simulink subsystem "AS_O2Input"  (R2022b)
settings: Solver=VariableStepAuto  StartTime=0.0  StopTime=10.0  RelTol=1e-3
undefined symbols (not defined in the file): O2_OutputDia
libraries: fl_lib x8, SimscapeFluids_lib x3, nesl_utility x3
settings Model: DefaultTestHarness=AS_O2Input_Test  Creator=CSN-Simulation  LastModifiedBy=MATLAB
settings DebuggingCC: UnconnectedInputMsg=warning  UnconnectedOutputMsg=warning  UnconnectedLineMsg=warning
settings ModelReferenceCC: EnableRefExpFcnMdlSchedulingChecks=on
settings RTWCC: DLArmComputeVersion=19.05

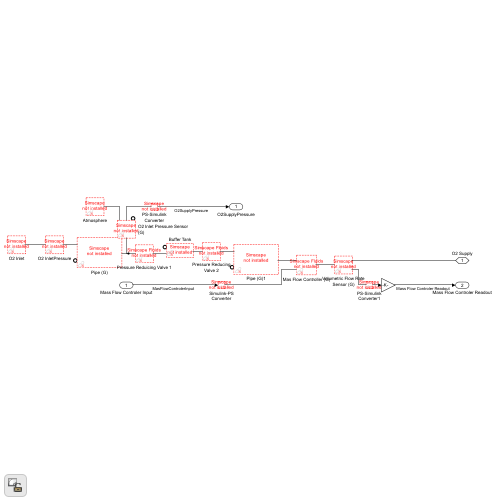
[thumbnail: Simulink's stored preview of the top-level diagram]
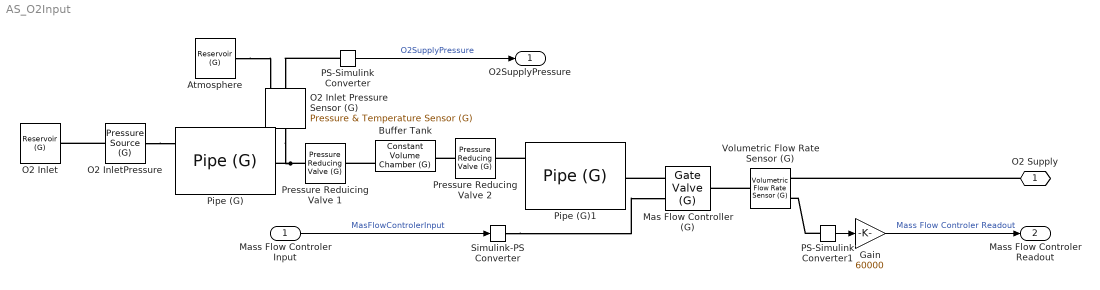
== system AS_O2Input ==
  Mass Flow Controler Input : Inport
  Atmosphere : fl_lib/Gas/Elements/Reservoir (G)  pressure_spec=foundation.enum.pressure_spec.atmospheric  reservoir_pressure=0.101325 MPa  reservoir_temperature=293.15 K  area_A=pi*(O2_OutputDia/2)^2 mm^2
  Buffer Tank : fl_lib/Gas/Elements/Constant Volume Chamber (G)  volume=O2_buffertank mm^3  num_ports=foundation.enum.num_ports.two  area_A=pi*(O2_OutputDia/2)^2 mm^2  area_B=pi*(O2_OutputDia/2)^2 mm^2  area_C=0.01 m^2  area_D=0.01 m^2  p_I_specify=off  p_I_priority=High  p_I=P_intermidiate Pa  p_I_nominal_specify=off  p_I_nominal_unit=MPa  p_I_nominal_value=1  T_I_specify=off  T_I_priority=High  T_I=T_room degC  T_I_nominal_specify=off  T_I_nominal_unit=K  T_I_nominal_value=1  rho_chamber_specify=off  rho_chamber_priority=None  rho_chamber=1.2 kg/m^3  rho_chamber_nominal_specify=off  rho_chamber_nominal_unit=kg/m^3  rho_chamber_nominal_value=1
      settings: InternalSimscapePortConfiguration="{\"Bottom\":[],\"Left\":[{\"id\":\"A\",\"label\":\"A\",\"type\":\"foundation.gas.gas\"},{\"id\":\"H\",\"label\":\"H\",\"type\":\"foundation.thermal.thermal\"}],\"Right\":[{\"id\":\"B\",\"label\":\"B\",\"type\":\"foundation.gas.gas\"}],\"Top\":[]}"
  Gain : Gain  Gain=60000
  Mas Flow Controller (G) : SimscapeFluids_lib/Gas/Valves & Orifices/Flow Control Valves/Gate Valve (G)  diam_orifice=O2_OutputDia-2 mm  x0=0  iso_cond_spec=fluids.gas.enum.flow_control_valve_spec.geometry  C_max=1.6 l/s/bar  B_crit=0.3  m=0.5  Cv_max=0.4  Kv_max=0.3  area_leak=1e-12 mm^2  area=pi*(O2_OutputDia/2)^2 mm^2  smoothing_factor=0  B_lam=0.999  T0=T_room degC  rho0=1.185 kg/m^3
      settings: InternalSimscapePortConfiguration="{\"Bottom\":[],\"Left\":[{\"id\":\"A\",\"label\":\"A\",\"type\":\"foundation.gas.gas\"},{\"id\":\"L\",\"label\":\"L\",\"type\":\"input\"}],\"Right\":[{\"id\":\"B\",\"label\":\"B\",\"type\":\"foundation.gas.gas\"}],\"Top\":[]}"
  O2 Inlet : fl_lib/Gas/Elements/Reservoir (G)  pressure_spec=foundation.enum.pressure_spec.atmospheric  reservoir_pressure=0.101325 MPa  reservoir_temperature=T_room degC  area_A=pi*(O2_OutputDia/2)^2 mm^2
  O2 Inlet Pressure Sensor (G) : fl_lib/Gas/Sensors/Pressure & Temperature Sensor (G)
      settings: InternalSimscapePortConfiguration="{\"Bottom\":[],\"Left\":[{\"id\":\"A\",\"label\":\"A\",\"type\":\"foundation.gas.gas\"}],\"Right\":[{\"id\":\"B\",\"label\":\"B\",\"type\":\"foundation.gas.gas\"},{\"id\":\"P\",\"label\":\"P\",\"type\":\"output\"},{\"id\":\"T\",\"label\":\"T\",\"type\":\"output\"}],\"Top\":[]}"
  O2 InletPressure : fl_lib/Gas/Sources/Pressure Source (G)  power_spec=foundation.enum.power_spec.isentropic  pressure_differential=P_inlet Pa  area_A=pi*(O2_OutputDia/2)^2 mm^2  area_B=pi*(O2_OutputDia/2)^2 mm^2
      settings: InternalSimscapePortConfiguration="{\"Bottom\":[],\"Left\":[{\"id\":\"A\",\"label\":\"A\",\"type\":\"foundation.gas.gas\"}],\"Right\":[{\"id\":\"B\",\"label\":\"B\",\"type\":\"foundation.gas.gas\"}],\"Top\":[]}"
  PS-Simulink Converter : nesl_utility/PS-Simulink Converter  PhysicalDomain=network_engine_domain  SubClassName=ps_output  LeftPortType=input  RightPortType=output  PseudoPeriodic=off  Frequencies=[]  Unit=Pa  AffineConversion=off
  PS-Simulink Converter1 : nesl_utility/PS-Simulink Converter  PhysicalDomain=network_engine_domain  SubClassName=ps_output  LeftPortType=input  RightPortType=output  PseudoPeriodic=off  Frequencies=[]  Unit=inherit  AffineConversion=off
  Pipe (G) : fl_lib/Gas/Elements/Pipe (G)  length=40 m  area=pi*(O2_OutputDia/2)^2 mm^2  Dh=O2_OutputDia mm  length_add=0.1 m  roughness=15e-6 m  Re_lam=2000  Re_tur=4000  shape_factor=64  Nu_lam=3.66  p_I_specify=off  p_I_priority=High  p_I=P_inlet Pa  p_I_nominal_specify=off  p_I_nominal_unit=MPa  p_I_nominal_value=1  T_I_specify=off  T_I_priority=High  T_I=293.15 K  T_I_nominal_specify=off  T_I_nominal_unit=K  T_I_nominal_value=1  rho_pipe_specify=off  rho_pipe_priority=None  rho_pipe=1.2 kg/m^3  rho_pipe_nominal_specify=off  rho_pipe_nominal_unit=kg/m^3  rho_pipe_nominal_value=1
  Pipe (G)1 : fl_lib/Gas/Elements/Pipe (G)  length=50 mm  area=pi*(O2_OutputDia/2)^2 mm^2  Dh=O2_OutputDia mm  length_add=0.1 m  roughness=15e-6 m  Re_lam=2000  Re_tur=4000  shape_factor=64  Nu_lam=3.66  p_I_specify=off  p_I_priority=High  p_I=0.101325 MPa  p_I_nominal_specify=off  p_I_nominal_unit=MPa  p_I_nominal_value=1  T_I_specify=off  T_I_priority=High  T_I=293.15 K  T_I_nominal_specify=off  T_I_nominal_unit=K  T_I_nominal_value=1  rho_pipe_specify=off  rho_pipe_priority=None  rho_pipe=1.2 kg/m^3  rho_pipe_nominal_specify=off  rho_pipe_nominal_unit=kg/m^3  rho_pipe_nominal_value=1
  Pressure Reducing Valve 2 : SimscapeFluids_lib/Gas/Valves & Orifices/Pressure Control Valves/Pressure Reducing Valve (G)  iso_cond_spec=fluids.gas.enum.iso_cond_spec.Kv  iso_opening_spec_C=fluids.gas.enum.iso_opening_spec.linear  p_set_gauge_C=0.1 MPa  p_range_C=0.1 MPa  C_max=1.6 l/s/bar  C_min=1e-5 l/s/bar  B_crit=0.3  p_control_C_TLU=[0.2 : 0.2 : 1.2] MPa  C_TLU=[1.6, 1.28, .96, .64, .32, 1e-05] l/s/bar  B_crit_TLU=0.3 * ones(1, 6)  m=0.5  iso_opening_spec_Cv=fluids.gas.enum.iso_opening_spec.linear  p_set_gauge_Cv=0.1 MPa  p_range_Cv=0.1 MPa  Cv_max=0.4  Cv_min=1e-6  p_control_Cv_TLU=[0.2 : 0.2 : 1.2] MPa  Cv_TLU=[.4, .32, .24, .16, .08, 1e-06]  iso_opening_spec_Kv=fluids.gas.enum.iso_opening_spec.linear  p_set_gauge_Kv=P_max_Gauge Pa  p_range_Kv=0.1 Pa  Kv_max=0.3  Kv_min=1e-6  p_control_Kv_TLU=[0.2 : 0.2 : 1.2] MPa  Kv_TLU=[.3, .24, .18, .12, .06, 1e-06]  iso_opening_spec_area=fluids.gas.enum.iso_opening_spec.linear  p_set_gauge_area=0.1 MPa  p_range_area=0.1 MPa  area_max=1e-4 m^2  area_leak=1e-12 m^2  p_control_area_TLU=[0.2 : 0.2 : 1.2] MPa  restriction_area_TLU=[1e-05, 8e-06, 6e-06, 4e-06, 2e-06, 1e-08] m^2  area=pi*(O2_OutputDia/2)^2 mm^2  smoothing_factor=0  B_lam=0.999  T0=T_room degC  rho0=1.185 kg/m^3
      settings: InternalSimscapePortConfiguration="{\"Bottom\":[],\"Left\":[{\"id\":\"A\",\"label\":\"A\",\"type\":\"foundation.gas.gas\"}],\"Right\":[{\"id\":\"B\",\"label\":\"B\",\"type\":\"foundation.gas.gas\"}],\"Top\":[]}"
  Pressure Reduicing Valve 1 : SimscapeFluids_lib/Gas/Valves & Orifices/Pressure Control Valves/Pressure Reducing Valve (G)  iso_cond_spec=fluids.gas.enum.iso_cond_spec.Kv  iso_opening_spec_C=fluids.gas.enum.iso_opening_spec.linear  p_set_gauge_C=0.1 MPa  p_range_C=0.1 MPa  C_max=1.6 l/s/bar  C_min=1e-5 l/s/bar  B_crit=0.3  p_control_C_TLU=[0.2 : 0.2 : 1.2] MPa  C_TLU=[1.6, 1.28, .96, .64, .32, 1e-05] l/s/bar  B_crit_TLU=0.3 * ones(1, 6)  m=0.5  iso_opening_spec_Cv=fluids.gas.enum.iso_opening_spec.linear  p_set_gauge_Cv=0.1 MPa  p_range_Cv=0.1 MPa  Cv_max=0.4  Cv_min=1e-6  p_control_Cv_TLU=[0.2 : 0.2 : 1.2] MPa  Cv_TLU=[.4, .32, .24, .16, .08, 1e-06]  iso_opening_spec_Kv=fluids.gas.enum.iso_opening_spec.linear  p_set_gauge_Kv=P_intermidiate Pa  p_range_Kv=0.1 Pa  Kv_max=0.3  Kv_min=1e-6  p_control_Kv_TLU=[0.2 : 0.2 : 1.2] MPa  Kv_TLU=[.3, .24, .18, .12, .06, 1e-06]  iso_opening_spec_area=fluids.gas.enum.iso_opening_spec.linear  p_set_gauge_area=0.1 MPa  p_range_area=0.1 MPa  area_max=1e-4 m^2  area_leak=1e-12 m^2  p_control_area_TLU=[0.2 : 0.2 : 1.2] MPa  restriction_area_TLU=[1e-05, 8e-06, 6e-06, 4e-06, 2e-06, 1e-08] m^2  area=pi*(O2_OutputDia/2)^2 mm^2  smoothing_factor=0  B_lam=0.999  T0=T_room degC  rho0=1.185 kg/m^3
      settings: InternalSimscapePortConfiguration="{\"Bottom\":[],\"Left\":[{\"id\":\"A\",\"label\":\"A\",\"type\":\"foundation.gas.gas\"}],\"Right\":[{\"id\":\"B\",\"label\":\"B\",\"type\":\"foundation.gas.gas\"}],\"Top\":[]}"
  Simulink-PS Converter : nesl_utility/Simulink-PS Converter  PhysicalDomain=network_engine_domain  SubClassName=ps_input  LeftPortType=input  RightPortType=output  PseudoPeriodic=off  Frequencies=[]  NoiseDistribution=none  NoiseParameters=[]  Unit=1  AffineConversion=off  FilteringAndDerivatives=provide  SimscapeFilterOrder=1  InputFilterTimeConstant=0.001  UdotUserProvided=0
  Volumetric Flow Rate Sensor (G) : fl_lib/Gas/Sensors/Volumetric Flow Rate Sensor (G)
      settings: InternalSimscapePortConfiguration="{\"Bottom\":[],\"Left\":[{\"id\":\"A\",\"label\":\"A\",\"type\":\"foundation.gas.gas\"}],\"Right\":[{\"id\":\"B\",\"label\":\"B\",\"type\":\"foundation.gas.gas\"},{\"id\":\"V\",\"label\":\"V\",\"type\":\"output\"}],\"Top\":[]}"
  O2 Supply : PMIOPort  Side=Right
  O2SupplyPressure : Outport
  Mass Flow Controler Readout : Outport  Port=2
  wires:
  Mass Flow Controler Input/1 -> Simulink-PS Converter/1  "MasFlowControlerInput"
  PS-Simulink Converter/1 -> O2SupplyPressure/1  "O2SupplyPressure"
  Gain/1 -> Mass Flow Controler Readout/1  "Mass Flow Controler Readout"
  PS-Simulink Converter1/1 -> Gain/1
  connections:
  O2 Inlet Pressure Sensor (G)/LConn1 -- Pipe (G)/RConn1 -- Pressure Reduicing Valve 1/LConn1
  Simulink-PS Converter/RConn1 -- Mas Flow Controller (G)/LConn2
  Atmosphere/LConn1 -- O2 Inlet Pressure Sensor (G)/RConn1
  O2 InletPressure/RConn1 -- Pipe (G)/LConn1
  PS-Simulink Converter/LConn1 -- O2 Inlet Pressure Sensor (G)/RConn2
  Mas Flow Controller (G)/LConn1 -- Pipe (G)1/RConn1
  Pipe (G)1/LConn1 -- Pressure Reducing Valve 2/RConn1
  Pressure Reducing Valve 2/LConn1 -- Buffer Tank/RConn1
  Buffer Tank/LConn1 -- Pressure Reduicing Valve 1/RConn1
  O2 InletPressure/LConn1 -- O2 Inlet/LConn1
  Volumetric Flow Rate Sensor (G)/LConn1 -- Mas Flow Controller (G)/RConn1
  O2 Supply/RConn1 -- Volumetric Flow Rate Sensor (G)/RConn1
  PS-Simulink Converter1/LConn1 -- Volumetric Flow Rate Sensor (G)/RConn2
